simulink model "Q10"  (R2016b)
settings: Solver=VariableStepAuto  StartTime=0.0  StopTime=10.0  RelTol=1e-3
settings Model: Creator=AKSHAY JP PAWAR  LastModifiedBy=AKSHAY JP PAWAR
settings DataIOCC: ReturnWorkspaceOutputs=on
settings SFSimCC: SimUseLocalCustomCode=on
settings RTWCC: RTWUseLocalCustomCode=on

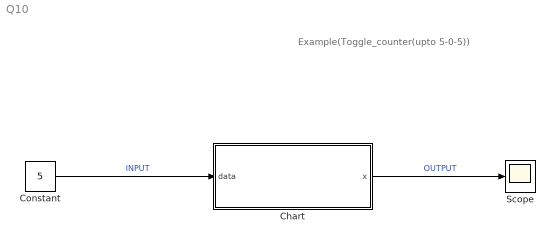
== system Q10 ==
  note: Example(Toggle_counter(upto 5-0-5))
  Chart : Stateflow chart  TreatAsAtomicUnit=on
  Constant : Constant  Value=5
  Scope : Scope
  wires:
  Constant/1 -> Chart/1(data)  "INPUT"
  Chart/1(x) -> Scope/1  "OUTPUT"

== stateflow chart Q10/Chart ==
  state Increasing
    en:
    x=0;
    during:
    x=x+1;
  state Decreasing
    during:
    x=x-1;
  (default) -> Increasing
  Increasing -> Decreasing : [x>=data]
  Decreasing -> Increasing : [x==0]
  data: data input; x output
